simulink model "U557E_MSM_PosSimDemo_2018b"  (R2018b)
settings: Solver=FixedStepAuto  StartTime=0.0  StopTime=5  FixedStep=0.01  RelTol=1e-3
libraries: simulink x1
settings Model: Creator=Louis  LastModifiedBy=szwsv4
settings DataIOCC: ReturnWorkspaceOutputs=on
settings OptimizationCC: DefaultParameterBehavior=Inlined  EnhancedBackFolding=on  PassReuseOutputArgsAs=Individual arguments  ZeroExternalMemoryAtStartup=off  ZeroInternalMemoryAtStartup=off  OptimizeBlockOrder=speed  DifferentSizesBufferReuse=on  OptimizationCustomize=off
settings DebuggingCC: ParameterTunabilityLossMsg=error
settings SFSimCC: SimAnalyzeCustomCode=on  MATLABDynamicMemAlloc=off
settings SFSimCC: SimCustomHeaderCode=|
  | #include "qmath.h"
  | #include "MsmInterfDet.h"
settings SFSimCC: SimUserSources=|
  | qmath.c
  | MsmInterfDet.c
settings RTWCC: SystemTargetFile=ert.tlc  TemplateMakefile=ert_default_tmf  RTWUseSimCustomCode=on
settings RTWCC: CustomHeaderCode=|
  | #include "qmath.h"
  | #include "MsmInterfDet.h"
settings RTWCC: CustomSource=|
  | qmath.c
  | MsmInterfDet.c
settings CodeAppCC: ForceParamTrailComments=on  IgnoreCustomStorageClasses=off  OperatorAnnotations=on  SimulinkDataObjDesc=on  SFDataObjDesc=on  InsertBlockDesc=on
settings ERTTargetCC: TargetLangStandard=C99 (ISO)  GenerateSampleERTMain=on  InlinedParameterPlacement=NonHierarchical  ERTCustomFileTemplate=example_file_process.tlc

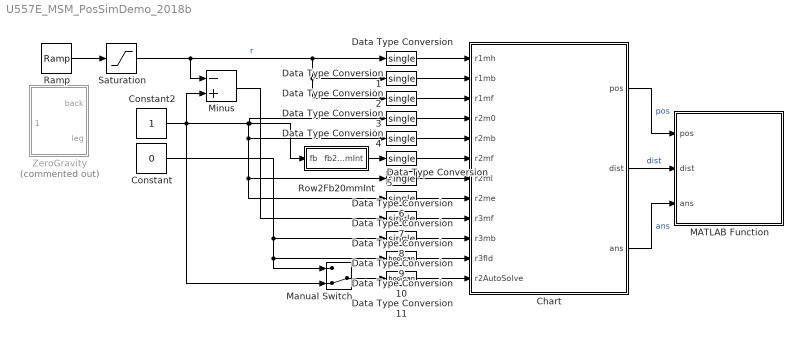
== system U557E_MSM_PosSimDemo_2018b ==
  Chart : Stateflow chart  TreatAsAtomicUnit=on
  Constant : Constant  Value=0
  Constant2 : Constant
  Data Type Conversion{,1..9} (10 alike) : DataTypeConversion  OutDataTypeStr=single  RndMeth=Simplest  SaturateOnIntegerOverflow=on
  Data Type Conversion10 : DataTypeConversion  OutDataTypeStr=boolean  RndMeth=Simplest  SaturateOnIntegerOverflow=on
  Data Type Conversion11 : DataTypeConversion  OutDataTypeStr=boolean  RndMeth=Simplest  SaturateOnIntegerOverflow=on
  MATLAB Function : MATLAB Function  TreatAsAtomicUnit=on
  Manual Switch : ManualSwitch  CurrentSetting=0
  Minus : Sum  Inputs=-+
  Ramp : simulink/Sources/Ramp  slope=1/5  start=0  InitialOutput=0
  Row2Fb20mmInt : Subsystem
  Saturation : Saturate  UpperLimit=1  LowerLimit=0
  ZeroGravity : Subsystem  Commented=on
  wires:
  Chart/1(pos) -> MATLAB Function/1(pos)  "pos"
  Saturation/1 -> Minus/1, Data Type Conversion2/1, Data Type Conversion1/1, Data Type Conversion/1  "r"
  Ramp/1 -> Saturation/1
  Data Type Conversion/1 -> Chart/1(r1mh)
  Data Type Conversion1/1 -> Chart/2(r1mb)
  Data Type Conversion2/1 -> Chart/3(r1mf)
  Data Type Conversion3/1 -> Chart/4(r2m0)
  Data Type Conversion4/1 -> Chart/5(r2mb)
  Data Type Conversion5/1 -> Chart/6(r2mf)
  Data Type Conversion6/1 -> Chart/7(r2ml)
  Data Type Conversion7/1 -> Chart/8(r2me)
  Data Type Conversion8/1 -> Chart/9(r3mf)
  Data Type Conversion9/1 -> Chart/10(r3mb)
  Data Type Conversion10/1 -> Chart/11(r3fld)
  Constant/1 -> Manual Switch/1, Data Type Conversion10/1, Data Type Conversion9/1
  Constant2/1 -> Row2Fb20mmInt/1(fb), Data Type Conversion3/1, Data Type Conversion7/1, Data Type Conversion6/1, Data Type Conversion4/1, Minus/2, Manual Switch/2
  Minus/1 -> Data Type Conversion8/1
  Data Type Conversion11/1 -> Chart/12(r2AutoSolve)
  Row2Fb20mmInt/1(fb20mmInt) -> Data Type Conversion5/1
  Manual Switch/1 -> Data Type Conversion11/1
  Chart/2(dist) -> MATLAB Function/2(dist)  "dist"
  Chart/3(ans) -> MATLAB Function/3(ans)  "ans"

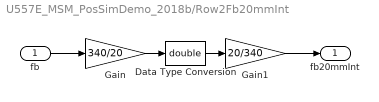
== system U557E_MSM_PosSimDemo_2018b/Row2Fb20mmInt ==
  fb : Inport
  Data Type Conversion : DataTypeConversion  OutDataTypeStr=double
  Gain : Gain  Gain=340/20  OutDataTypeStr=uint16  RndMeth=Round  SaturateOnIntegerOverflow=on
  Gain1 : Gain  Gain=20/340  RndMeth=Round  SaturateOnIntegerOverflow=on
  fb20mmInt : Outport
  wires:
  Gain1/1 -> fb20mmInt/1
  Data Type Conversion/1 -> Gain1/1
  Gain/1 -> Data Type Conversion/1
  fb/1 -> Gain/1

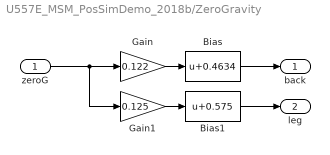
== system U557E_MSM_PosSimDemo_2018b/ZeroGravity ==
  zeroG : Inport
  Bias : Bias  Bias=0.4634
  Bias1 : Bias  Bias=0.575
  Gain : Gain  Gain=0.122
  Gain1 : Gain  Gain=0.125
  back : Outport
  leg : Outport  Port=2
  wires:
  Bias/1 -> back/1
  zeroG/1 -> Gain/1, Gain1/1
  Bias1/1 -> leg/1
  Gain1/1 -> Bias1/1
  Gain/1 -> Bias/1

== matlab function U557E_MSM_PosSimDemo_2018b/MATLAB Function ==
  data: pos input; dist input; ans input
function ShowMsmSeats(pos,dist,ans)
eml.extrinsic('plot','text');%声明不能生成c代码的函数

hold off;
plot([pos.GT1.x;pos.GT2.x],[pos.GT1.z;pos.GT2.z],'k');
hold on;
axis equal;
topleft=[2600;1750];
xlim([topleft(1),6000]);
ylim([500,topleft(2)]);

DrawDraft(pos.seat,pos.r3fld);

plot([pos.GT2.x;pos.GT3.x],[pos.GT2.z;pos.GT3.z],'k');
plot([pos.GT2.x;pos.GT4.x],[pos.GT2.z;pos.GT4.z],'k');
plot([pos.GT4.x;pos.GT5.x],[pos.GT4.z;pos.GT5.z],'k');
plot([pos.GT5.x;pos.GT6.x],[pos.GT5.z;pos.GT6.z],'k');
plot([pos.GT5.x;pos.GT3.x],[pos.GT5.z;pos.GT3.z],'k');
plot([pos.GT1.x;pos.GT6.x],[pos.GT1.z;pos.GT6.z],'k');
plot([pos.GT3.x;pos.p1_bkAxis.x],[pos.GT3.z;pos.p1_bkAxis.z],'k');
plot([pos.p1_bkSdUp.x;pos.p1_bkSdMd.x],[pos.p1_bkSdUp.z;pos.p1_bkSdMd.z],'k');
plot([pos.p1_bkSdDwn.x;pos.p1_bkSdMd.x],[pos.p1_bkSdDwn.z;pos.p1_bkSdMd.z],'k');
plot([pos.p1_bkUp.x;pos.p1_bkMd.x],[pos.p1_bkUp.z;pos.p1_bkMd.z],'k');
plot([pos.p1_bkDwn.x;pos.p1_bkMd.x],[pos.p1_bkDwn.z;pos.p1_bkMd.z],'k');
plot(pos.GT6.x,pos.GT6.z,'ro');
text(double(pos.GT6.x),double(pos.GT6.z),"\Leftarrow Hight"+round(pos.req_r1mh*100)+"%");
plot(pos.GT5.x,pos.GT5.z,'rx');
text(double(pos.GT5.x),double(pos.GT5.z),"\Leftarrow Fwd/Bwd"+round(pos.req_r1mf*100)+"%");
plot(pos.p1_bkAxis.x,pos.p1_bkAxis.z,'ro');
text(double(pos.p1_bkAxis.x),double(pos.p1_bkAxis.z),"\Leftarrow Back"+round(pos.req_r1mb*100)+"%");

plot([pos.LY1.x;pos.LY2.x],[pos.LY1.z;pos.LY2.z],'m');
plot([pos.LY3.x;pos.LY2.x],[pos.LY3.z;pos.LY2.z],'m');
plot([pos.LY3.x;pos.LY4.x],[pos.LY3.z;pos.LY4.z],'m');
plot([pos.LY1.x;pos.LY4.x],[pos.LY1.z;pos.LY4.z],'m');
plot(pos.p2_Scrn.x,pos.p2_Scrn.z,'mx');
plot(pos.p2_LgRstAxis.x,pos.p2_LgRstAxis.z,'mo');
plot([pos.p2_LgRstA.x;pos.p2_LgRstB.x],[pos.p2_LgRstA.z;pos.p2_LgRstB.z],'m');
plot([pos.p2_LgRstC.x;pos.p2_LgRstB.x],[pos.p2_LgRstC.z;pos.p2_LgRstB.z],'m');
plot([pos.p2_LgRstC.x;pos.p2_LgRstD.x],[pos.p2_LgRstC.z;pos.p2_LgRstD.z],'m');
plot(pos.p2_bkAxis.x,pos.p2_bkAxis.z,'mo');
plot([pos.p2_bkUp.x;pos.p2_bkDwn.x],[pos.p2_bkUp.z;pos.p2_bkDwn.z],'m');
plot([pos.pg_a.x;pos.pg_b.x],[pos.pg_a.z;pos.pg_b.z],'b');
plot(pos.LY2.x,pos.LY2.z,'ro');
if ans.ans_get>0
text(double(pos.LY2.x),double(pos.LY2.z),"\Leftarrow 0 Gravity"+round(ans.ans_r2m0*100)+"%");
plot(pos.LY1.x,pos.LY1.z,'rx');
text(double(pos.LY1.x),double(pos.LY1.z),"\Leftarrow Fwd/Bwd"+round(ans.ans_r2mf*100)+"%");
plot(pos.p2_bkAxis.x,pos.p2_bkAxis.z,'ro');
text(double(pos.p2_bkAxis.x),double(pos.p2_bkAxis.z),"\Leftarrow Back"+round(ans.ans_r2mb*100)+"%");
plot(pos.p2_LgRstAxis.x,pos.p2_LgRstAxis.z,'ro');
text(double(pos.p2_LgRstAxis.x),double(pos.p2_LgRstAxis.z),"\Leftarrow Leg Rest"+round(ans.ans_r2ml*100)+"%");
plot(pos.p2_LgRstC.x,pos.p2_LgRstC.z,'rx');
text(double(pos.p2_LgRstC.x),double(pos.p2_LgRstC.z),"\Leftarrow Leg Ext"+round(ans.ans_r2me*100)+"%");
else
text(double(pos.LY2.x),double(pos.LY2.z),"\Leftarrow 0 Gravity"+round(pos.req_r2m0*100)+"%");
plot(pos.LY1.x,pos.LY1.z,'rx');
text(double(pos.LY1.x),double(pos.LY1.z),"\Leftarrow Fwd/Bwd"+round(pos.req_r2mf*100)+"%");
plot(pos.p2_bkAxis.x,pos.p2_bkAxis.z,'ro');
text(double(pos.p2_bkAxis.x),double(pos.p2_bkAxis.z),"\Leftarrow Back"+round(pos.req_r2mb*100)+"%");
plot(pos.p2_LgRstAxis.x,pos.p2_LgRstAxis.z,'ro');
text(double(pos.p2_LgRstAxis.x),double(pos.p2_LgRstAxis.z),"\Leftarrow Leg Rest"+round(pos.req_r2ml*100)+"%");
plot(pos.p2_LgRstC.x,pos.p2_LgRstC.z,'rx');
text(double(pos.p2_LgRstC.x),double(pos.p2_LgRstC.z),"\Leftarrow Leg Ext"+round(pos.req_r2me*100)+"%");
end

plot(pos.p3_seat.x,pos.p3_seat.z,'kx');
plot(pos.p3_bkAxis.x,pos.p3_bkAxis.z,'ko');
if pos.seat==7
    plot(pos.p3_seatAxis.x,pos.p3_seatAxis.z,'ko');
    plot([pos.p3_seat.x;pos.p3_seatAxis.x],[pos.p3_seat.z;pos.p3_seatAxis.z],'k');
    if pos.r3fld>0
        plot([pos.p3_pillowF.x;pos.p3_pillowB.x],[pos.p3_pillowF.z;pos.p3_pillowB.z],'k');
        plot([pos.p3_seatAxis.x;pos.p3_pillowB.x],[pos.p3_seatAxis.z;pos.p3_pillowB.z],'k');
    else
        plot([pos.p3_bkUp.x;pos.p3_bkDwn.x],[pos.p3_bkUp.z;pos.p3_bkDwn.z],'k');
    end
else
    plot([pos.p3_seat.x;pos.p3_bkAxis.x],[pos.p3_seat.z;pos.p3_bkAxis.z],'k');
    plot([pos.p3_bkUp.x;pos.p3_bkDwn.x],[pos.p3_bkUp.z;pos.p3_bkDwn.z],'k');
end
text(double(pos.p3_bkAxis.x),double(pos.p3_bkAxis.z),"\Leftarrow Back"+round(pos.req_r3mb*100)+"%");    
text(double(pos.p3_seat.x),double(pos.p3_seat.z),"\Leftarrow Fwd/Bwd"+round(pos.req_r3mf*100)+"%");

plot(pos.p4.x,pos.p4.z,'bx');

draw=1;
%check row1 and row2
pd_scrn1=GetDrawPedal(draw,pt2col(pos.p2_Scrn),pt2col(pos.p1_bkSdMd),pt2col(pos.p1_bkSdUp),0);
pd_scrn2=GetDrawPedal(draw,pt2col(pos.p2_Scrn),pt2col(pos.p1_bkSdDwn),pt2col(pos.p1_bkSdMd),0);
d1s=min(pd_scrn1,pd_scrn2);

pd_LgRstA1=GetDrawPedal(draw,pt2col(pos.p2_LgRstA),pt2col(pos.p1_bkDwn),pt2col(pos.p1_bkMd),0);
pd_LgRstB1=GetDrawPedal(draw,pt2col(pos.p2_LgRstB),pt2col(pos.p1_bkDwn),pt2col(pos.p1_bkMd),0);
pd_LgRstC1=GetDrawPedal(draw,pt2col(pos.p2_LgRstC),pt2col(pos.p1_bkDwn),pt2col(pos.p1_bkMd),0);
pd_LgRstA2=GetDrawPedal(draw,pt2col(pos.p2_LgRstA),pt2col(pos.p1_bkMd),pt2col(pos.p1_bkUp),0);
pd_LgRstB2=GetDrawPedal(draw,pt2col(pos.p2_LgRstB),pt2col(pos.p1_bkMd),pt2col(pos.p1_bkUp),0);
pd_LgRstC2=GetDrawPedal(draw,pt2col(pos.p2_LgRstC),pt2col(pos.p1_bkMd),pt2col(pos.p1_bkUp),0);
R2LgA_R1Bk=min(pd_LgRstA1,pd_LgRstA2);
R2LgB_R1Bk=min(pd_LgRstB1,pd_LgRstB2);
R2LgC_R1Bk=min(pd_LgRstC1,pd_LgRstC2);
d1l=min(min(R2LgA_R1Bk,R2LgB_R1Bk),R2LgC_R1Bk);

%check row2 and row3
if pos.seat==7 && pos.r3fld>0
    pd_p3_pillowF=GetDrawPedal(draw,pt2col(pos.p3_pillowF),pt2col(pos.p2_bkDwn),pt2col(pos.p2_bkUp),1);
    pd_p3_pillowB=GetDrawPedal(draw,pt2col(pos.p3_pillowB),pt2col(pos.p2_bkDwn),pt2col(pos.p2_bkUp),1);
    d2=min(pd_p3_pillowF,pd_p3_pillowB);
    d3=9999;
else
    d2=GetDrawPedal(draw,pt2col(pos.p3_seat),pt2col(pos.p2_bkDwn),pt2col(pos.p2_bkUp),1);
    d3=GetDrawPedal(draw,pt2col(pos.p4),pt2col(pos.p3_bkDwn),pt2col(pos.p3_bkUp),0);
end


if pos.seat==7
    d3f=GetDrawPedal(draw,pt2col(pos.p3_seatAxis),pt2col(pos.p2_bkDwn),pt2col(pos.p2_bkUp),1);
else
    d3f=9999;
end

text(topleft(1)+20,topleft(2)-50,"d1l:"+round(dist.d1l)+";d1s:"+round(dist.d1s)+";d2:"+round(dist.d2)+":d3:"+round(dist.d3)+";d3f:"+round(dist.d3f));
end

function r=pt2col(x)
    r=[double(x.x);0;double(x.z)];
end

function DrawDraft(seat,r3fld)
persistent ShowMsmSeatsInitd;
persistent GT1_0 GT2_0 GT3_0 GT4_0 GT5_0 GT6_0 GT1_100 GT2_100 GT3_100 GT4_100 GT5_100 GT6_100 p1_bkAxis_0 p1_bkAxis_100;
persistent p1_bkSdUp_0 p1_bkSdMd_0 p1_bkSdDwn_0 p1_bkSdUp_100 p1_bkSdMd_100 p1_bkSdDwn_100;
persistent p1_bkUp_0 p1_bkMd_0 p1_bkDwn_0 p1_bkUp_100 p1_bkMd_100 p1_bkDwn_100;
persistent LY1_0 LY2_0 LY3_0 LY4_0 LY1_100 LY2_100 LY3_100 LY4_100;
persistent p2_Scrn_0 p2_Scrn_100;
persistent p2_LgRstAxis_f0g0 p2_LgRstA_f0g0 p2_LgRstAxis_f1g1 p2_LgRstA_f1g1;
persistent p2_LgRstB_f0r0e0g0 p2_LgRstC_f0r0e0g0 p2_LgRstD_f0r0e0g0;
persistent p2_LgRstB_f1r1e1g1 p2_LgRstC_f1r1e1g1 p2_LgRstD_f1r1e1g1;
persistent p2_LgRstAxis_f1g0 p2_LgRstA_f1g0 p2_LgRstB_f1r1e1g0 p2_LgRstC_f1r1e1g0 p2_LgRstD_f1r1e1g0;
persistent p2_bkAxis_0 p2_bkAxis_100_z0 p2_bkAxis_100_z15 p2_bkUp_0 p2_bkUp_100_z15 p2_bkDwn_0 p2_bkDwn_100_z15;
persistent p4 pg_a pg_b;
persistent p3_seat_0 p3_seat_100;
persistent p3_bkUp_0 p3_bkDwn_0 p3_bkAxis_0;
persistent p3_bkUp_100 p3_bkDwn_100 p3_bkAxis_100;
persistent p3_seatAxis_0 p3_seatAxis_100 p3_pillowF_0 p3_pillowB_0 p3_pillowF_100 p3_pillowB_100;

if isempty(ShowMsmSeatsInitd)
    GT1_0=[2678.3150;0;788.0193];
    GT2_0=[2775.7968;0;786.0415];
    GT3_0=[3052.8180;0;745.4054];
    GT4_0=[2678.5577;0;746.5067];
    GT5_0=[2951.4735;0;733.8440];
    GT6_0=[2955.3233;0;700.0519];
    GT1_100=[2906.5401;0;819.5478];
    GT2_100=[3003.9375;0;824.059];
    GT3_100=[3283.0483;0;801.9408];
    GT4_100=[2938.5181;0;741.9691];
    GT5_100=[3211.4339;0;729.3064];
    GT6_100=[3235.6489;0;705.4242];
    p1_bkAxis_0=[3083.9187;0;833.6201];
    p1_bkAxis_100=[3308.2119;0;892.029];
    p1_bkSdUp_0=[3030.1468;0;1473.1297];
    p1_bkSdMd_0=[3115.3845;0;1341.5191];
    p1_bkSdDwn_0=[3119.0948;0;945.0812];
    p1_bkSdUp_100=[3860.49;0;1218.9125];
    p1_bkSdMd_100=[3779.1299;0;1084.8701];
    p1_bkSdDwn_100=[3423.8680;0;908.8993];
    p1_bkUp_0=[3095.9513;0;1515.7480];
    p1_bkMd_0=[3192.1518;0;1367.2105];
    p1_bkDwn_0=[3156.1095;0;692.3232];
    p1_bkUp_100=[3927.5104;0;1178.2329];
    p1_bkMd_100=[3835.6862;0;1026.9509];
    p1_bkDwn_100=[3212.4507;0;765.5137];

    LY1_0=[4013.5391;0;751.8094;1];
    LY2_0=[3766.5088;0;754.4203;1];
    LY3_0=[3675.6638;0;763.2210;1];
    LY4_0=[3786.2759;0;809.7597;1];
    LY1_100=[4353.0329;0;770.3569;1];
    LY2_100=[4106.0026;0;772.9677;1];
    LY3_100=[4039.3464;0;835.3154;1];
    LY4_100=[4148.5119;0;885.1527;1];
    p2_Scrn_0=[3607.8959;0;1118.4741;1];
    p2_Scrn_100=[3947.3896;0;1137.0216;1];
    p2_LgRstAxis_f0g0=[3595.2251;0;905.0559;1];
    p2_LgRstA_f0g0=[3620.2973;0;933.766;1];
    p2_LgRstB_f0r0e0g0=[3537.8699;0;869.4523;1];
    p2_LgRstC_f0r0e0g0=[3539.5585;0;584.4573;1];
    p2_LgRstD_f0r0e0g0=[3599.5585;0;584.4573;1];
    p2_LgRstAxis_f1g1=[3988.6367;0;1026.6492;1];
    p2_LgRstA_f1g1=[4020.2853;0;1047.8919;1];
    p2_LgRstB_f1r1e1g1=[3742.5588;0;1097.9077;1];
    p2_LgRstC_f1r1e1g1=[3458.5168;0;1121.2561;1];
    p2_LgRstD_f1r1e1g1=[3453.2472;0;1061.4897;1];
    p2_LgRstAxis_f1g0=[3934.7188;0;923.6033;1];
    p2_LgRstA_f1g0=[3959.791;0;952.3134;1];
    p2_LgRstB_f1r1e1g0=[3678.5828;0;928.7441;1];
    p2_LgRstC_f1r1e1g0=[3398.1763;0;877.7814;1];
    p2_LgRstD_f1r1e1g0=[3408.5553;0;818.6859;1];
    p2_bkUp_0=[4201.24591;0;1443.0824;1];
    p2_bkDwn_0=[4186.8594;0;1068.2653;1];
    p2_bkAxis_0=[4138.065;0;859.628;1];
    p2_bkUp_100_z15=[5073.267;0;709.1434;1];
    p2_bkDwn_100_z15=[4702.997;0;769.1015;1];
    p2_bkAxis_100_z15=[4502.187;0;842.0132;1];
    p2_bkAxis_100_z0=Trans(LY1_100-LY1_0)*hmg(p2_bkAxis_0);

    pg_a=[3318.556;0;554.144;1];
    pg_b=[4037.4839;0;593.42;1];

    %7 seats configuraiton only
    p3_seatAxis_0=[4923.4164;0;980.9009;1];%OTF
    p3_seatAxis_100=[5253.4164;0;980.9009;1];%OTF
    p3_pillowF_0=[4042.3140;0;854.6288;1];%OTF
    p3_pillowB_0=[4020.0008;0;959.8990;1];%OTF
	p3_pillowF_100=Trans(p3_seatAxis_100-p3_seatAxis_0)*hmg(p3_pillowF_0);
    p3_pillowB_100=Trans(p3_seatAxis_100-p3_seatAxis_0)*hmg(p3_pillowB_0);
    if seat==6
        p3_seat_0=[4462.1043;0;989.4298;1];
        p3_seat_100=[4792.1043;0;989.4298;1];
        p3_bkUp_0=[4900.2;0;1723.11;1];
        p3_bkDwn_0=[5109.58;0;1412.38;1];
        p3_bkAxis_0=[5011.46;0;919.75;1];
        p3_bkUp_100=[5945.25;0;1461.23;1];
        p3_bkDwn_100=[5804.74;0;1113.89;1];
        p3_bkAxis_100=[5341.46;0;919.45;1];
    else%if seat==7
        p3_seat_0=[4485.6458;0;978.1299;1];
        p3_seat_100=[4815.6458;0;978.1299;1];
        p3_bkUp_0=[5131.29;0;1690.95;1];
        p3_bkDwn_0=[5102.69;0;1281.95;1];
        p3_bkAxis_0=[5022.3;0;905.73;1];
        p3_bkUp_100=[5976.16;0;1394.86;1];
        p3_bkDwn_100=[5671.47;0;1120.52;1];
        p3_bkAxis_100=[5352.3;0;905.73;1];
    end

    p4=[5765.1;0;1350.88;1];
    ShowMsmSeatsInitd=int32(seat);
end

pyp(GT1_0,GT2_0,'c');pyp(GT1_100,GT2_100,'c');
pyp(GT2_0,GT3_0,'c');pyp(GT2_100,GT3_100,'c');
pyp(GT3_0,p1_bkAxis_0,'c');pyp(GT3_100,p1_bkAxis_100,'c');
pyp(GT3_0,GT5_0,'c');pyp(GT3_100,GT5_100,'c');
pyp(GT2_0,GT4_0,'c');pyp(GT2_100,GT4_100,'c');
pyp(GT4_0,GT5_0,'c');pyp(GT4_100,GT5_100,'c');
pyp(GT5_0,GT6_0,'c');pyp(GT5_100,GT6_100,'c');
pyp(GT1_0,GT6_0,'c');pyp(GT1_100,GT6_100,'c');
pyp(p1_bkSdMd_0,p1_bkSdUp_0,'c');pyp(p1_bkSdMd_100,p1_bkSdUp_100,'c');
pyp(p1_bkSdMd_0,p1_bkSdDwn_0,'c');pyp(p1_bkSdMd_100,p1_bkSdDwn_100,'c');
pyp(p1_bkMd_0,p1_bkUp_0,'c');pyp(p1_bkMd_100,p1_bkUp_100,'c');
pyp(p1_bkMd_0,p1_bkDwn_0,'c');pyp(p1_bkMd_100,p1_bkDwn_100,'c');

pyp(LY1_0,LY2_0,'c');pyp(LY2_0,LY3_0,'c');pyp(LY3_0,LY4_0,'c');pyp(LY4_0,LY1_0,'c');
pyp(LY1_100,LY2_100,'c');pyp(LY2_100,LY3_100,'c');pyp(LY3_100,LY4_100,'c');pyp(LY4_100,LY1_100,'c');
pyd(p2_Scrn_0,'cx');pyd(p2_Scrn_100,'cx');
pyd(p2_LgRstAxis_f0g0,'co');pyd(p2_LgRstAxis_f1g0,'co');pyd(p2_LgRstAxis_f1g1,'co');
pyp(p2_LgRstA_f0g0,p2_LgRstB_f0r0e0g0,'c');pyp(p2_LgRstB_f0r0e0g0,p2_LgRstC_f0r0e0g0,'c');pyp(p2_LgRstC_f0r0e0g0,p2_LgRstD_f0r0e0g0,'c');
pyp(p2_LgRstA_f1g1,p2_LgRstB_f1r1e1g1,'c');pyp(p2_LgRstB_f1r1e1g1,p2_LgRstC_f1r1e1g1,'c');pyp(p2_LgRstC_f1r1e1g1,p2_LgRstD_f1r1e1g1,'c');
pyp(p2_LgRstA_f1g0,p2_LgRstB_f1r1e1g0,'c');pyp(p2_LgRstB_f1r1e1g0,p2_LgRstC_f1r1e1g0,'c');pyp(p2_LgRstC_f1r1e1g0,p2_LgRstD_f1r1e1g0,'c');
pyd(p2_bkAxis_0,"co");
pyd(p2_bkAxis_100_z0,"co");
pyd(p2_bkAxis_100_z15,"co");
pyp(p2_bkUp_0,p2_bkDwn_0,'c');
pyp(p2_bkUp_100_z15,p2_bkDwn_100_z15,'c');
pyp(pg_a,pg_b,'c');

pyd(p3_seat_0,'cx');
pyp(p3_bkUp_0,p3_bkDwn_0,'c');
pyd(p3_bkAxis_0,'co');
pyp(p3_bkUp_100,p3_bkDwn_100,'c');
pyd(p3_bkAxis_100,'co');
pyd(p3_seat_100,'cx');
if seat==7
    pyd(p3_seatAxis_0,'co');
    pyp(p3_seatAxis_0,p3_seat_0,'c');
    pyd(p3_seatAxis_100,'co');
    pyp(p3_seatAxis_100,p3_seat_100,'c');
    if r3fld>0
        pyp(p3_seatAxis_0,p3_pillowB_0,'c');
        pyp(p3_seatAxis_100,p3_pillowB_100,'c');
        pyp(p3_pillowF_0,p3_pillowB_0,'c');
        pyp(p3_pillowF_100,p3_pillowB_100,'c');
    end
else
    pyp(p3_seat_0,p3_bkAxis_0,'c');
    pyp(p3_seat_100,p3_bkAxis_100,'c');
end

end
function r=Sat(n,lo,hi)
    if n<=lo
        r=lo;
    elseif n>=hi
        r=hi;
    else
        r=n;
    end
end

function r=solveLinkMid(A,B,MA,MB)
x1=A(1);y1=A(3);r1=MA;
x2=B(1);y2=B(3);r2=MB;
x1_2=x1^2;
y1_2=y1^2;
r1_2=r1^2;
D1=-2*x1;F1=x1_2+y1_2-r1_2;
a=(y1-y2)/(x2-x1);
b=(x2^2+y2^2-r2^2-x1_2-y1_2+r1_2)/(2*(x2-x1));
AA=a^2+1;
BB=2*a*b+D1*a-2*y1;
CC=b^2+D1*b+F1;
s=sqrt(BB^2-4*AA*CC);
y1=(-BB+s)/(2*AA);y2=(-BB-s)/(2*AA);
x1=a*y1+b;x2=a*y2+b;
r=[x1,x2;0,0;y1,y2;1,1];
end
function pyp(a,b,p)
plot([a(1);b(1)],[a(3);b(3)],p);
end
function py(a,b)
plot([a(1);b(1)],[a(3);b(3)],'k');
end
function pyd(a,s)
plot(a(1),a(3),s);
end
function r=d(a,b)
r=sqrt((a(1)-b(1))^2+(a(2)-b(2))^2+(a(3)-b(3))^2);
end

function r=RotX(t)
r=[...
1,0,0,0;...
0,cos(t),-sin(t),0;...
0,sin(t),cos(t),0;
0,0,0,1];
end
function r=RotY(t)
r=[...
cos(t),0,sin(t),0;...
0,1,0,0;...
-sin(t),0,cos(t),0;...
0,0,0,1];
end
function r=RotZ(t)
r=[...
cos(t),-sin(t),0,0;...
sin(t),cos(t),0,0;...
0,0,1,0;...
0,0,0,1];
end
function r=vers(t)
r=1-cos(t);
end
function r=Rot(A,t)
k=unit([0;0;0;1],A);
r=[...
k(1)*k(1)*vers(t)+cos(t),k(2)*k(1)*vers(t)-k(3)*sin(t),k(3)*k(1)*vers(t)+k(2)*sin(t),0;...
k(1)*k(2)*vers(t)+k(3)*sin(t),k(2)*k(2)*vers(t)+cos(t),k(3)*k(2)*vers(t)-k(1)*sin(t),0;...
k(1)*k(3)*vers(t)-k(2)*sin(t),k(2)*k(3)*vers(t)+k(1)*sin(t),k(3)*k(3)*vers(t)+cos(t),0;...
0,0,0,1];
end
function r=unit(A,B)
m=d(A,B);
v=B-A;
r=[v(1)/m;v(2)/m;v(3)/m;1];
end
function r=Trans(A)
r=[...
1,0,0,A(1);...
0,1,0,A(2);...
0,0,1,A(3);...
0,0,0,1];
end
function r=hmg(A)%homogeneous
r=[A(1);A(2);A(3);1];
end
function r=AngleInc(A,B)
r=acos((A(1)*B(1)+A(2)*B(2)+A(3)*B(3))/(d(A,[0;0;0])*d(B,[0;0;0])));
r=real(r);
end
function r=Mid(A,B)
r=[(A(1)+B(1))/2;(A(2)+B(2))/2;(A(3)+B(3))/2;1];
end
function [r,in]=GetPedal(D,A,B)
    dx=A(1)-B(1);
    dy=A(2)-B(2);
    dz=A(3)-B(3);
    u=(D(1)-A(1))*dx+(D(2)-A(2))*dy+(D(3)-A(3))*dz;
    u=u/(dx^2+dy^2+dz^2);
    r=[A(1)+u*dx;A(2)+u*dy;A(3)+u*dz;1];
    in=0;
    if ((A(1)<=B(1) && r(1)>=A(1) && r(1)<=B(1))||(B(1)<=A(1) && r(1)>=B(1) && r(1)<=A(1)))...
    && ((A(2)<=B(2) && r(2)>=A(2) && r(2)<=B(2))||(B(2)<=A(2) && r(2)>=B(2) && r(2)<=A(2)))...
    && ((A(3)<=B(3) && r(3)>=A(3) && r(3)<=B(3))||(B(3)<=A(3) && r(3)>=B(3) && r(3)<=A(3)))
        in=1;
    end
end
function r=GetDrawPedal(draw,D,A,B,ext)
    r=9999;
    [pd,in]=GetPedal(D,A,B);
    da=d(pd,A);
    db=d(pd,B);
    if in>0 || ext
        r=d(pd,D);
        if draw>0
            pyp(pd,D,'k:');
        end
        dd=Mid(pd,D);
        if pd(1)>D(1)...
        || (pd(3)>D(3) && A(1)>B(1) && A(3)>B(3))...
        || (pd(3)<D(3) && A(1)<B(1) && A(3)>B(3))
            r=-r;
            if draw>0
                text(dd(1),dd(3),""+round(r),'Color','red');
            end
        else
            if draw>0
                text(dd(1),dd(3),""+round(r),'Color','blue');
            end
        end
        if ext && draw>0
            if da<db
                pyp(pd,A,'k:');
            else
                pyp(pd,B,'k:');
            end
        end
    else
        if da<db
            r=d(A,D);
            dd=Mid(A,D);
            if draw>0
                pyp(A,D,'k:');
                text(dd(1),dd(3),""+round(r),'Color','green');
            end
        else
            r=d(B,D);
            dd=Mid(B,D);
            if draw>0
                pyp(B,D,'k:');
                text(dd(1),dd(3),""+round(r),'Color','green');
            end
        end

    end
end

== stateflow chart U557E_MSM_PosSimDemo_2018b/Chart ==
  (default) -> (junction 19)
  (junction 19) -> (junction 25) [order 2]
  (junction 25) -> (junction 24)
  (junction 19) -> (junction 21) [order 1] : [r2AutoSolve && ...
      | MsmInterfDet_WisdomEnjoySearch(7,r1mh,r1mb,r1mf,r3mf)>0]
      | {ans=MsmInterfDet_GetAns();
      | MsmInterfDet_Upd(7,r1mh,r1mb,r1mf, ans.ans_r2m0,ans.ans_r2mb,ans.ans_r2mf,ans.ans_r2ml,ans.ans_r2me, r3mf,r3mb,r3fld);
      | pos=MsmInterfDet_GetPos();
      | dist=MsmInterfDet_GetInterf();}
  (junction 24) -> (junction 21) : {MsmInterfDet_Upd(7,r1mh,r1mb,r1mf, r2m0,r2mb,r2mf,r2ml,r2me, r3mf,r3mb,r3fld);
      | pos=MsmInterfDet_GetPos();
      | dist=MsmInterfDet_GetInterf();}
  data: pos output Bus: MsmPosTyp; r1mh input single; r1mb input single; r1mf input single; r2m0 input single; r2mb input single; r2mf input single; r2ml input single; r2me input single; r3mf input single; r3mb input single; r3fld input boolean; r2AutoSolve input boolean; dist output Bus: MsmDistTyp; ans output Bus: MsmAnsTyp
